simulink model "First_Model"  (R2021b)
settings: Solver=VariableStepDiscrete  StartTime=0.0  StopTime=200  MaxStep=inf  RelTol=1e-3
undefined symbols (not defined in the file): f, m, n
settings Model: Creator=david  LastModifiedBy=andry
settings SolverCC: AlgebraicLoopSolver=TrustRegion
settings DebuggingCC: SFMachineParentedDataDiag=warning

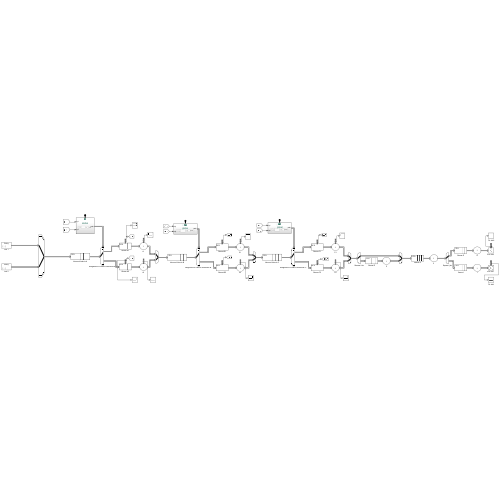
[thumbnail: Simulink's stored preview of the top-level diagram]
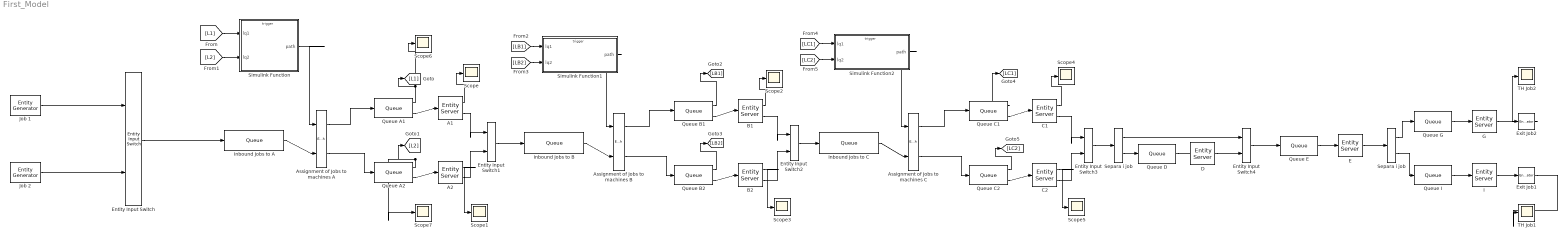
== system First_Model ==
  A1 : EntityServer  InputPortMessageModes=m  OutputPortMessageModes=n,m  Capacity=1  ServiceTimeValue=3  NumberEntitiesDeparted=on
      settings: OutputPortMap=o0,o9
  A2 : EntityServer  InputPortMessageModes=m  OutputPortMessageModes=n,m  Capacity=1  ServiceTimeValue=3  NumberEntitiesDeparted=on
      settings: OutputPortMap=o0,o9
  Assignment of Jobs to machines A : EntityOutputSwitch  InputPortMessageModes=m,m  OutputPortMessageModes=m,m  SwitchingCriterion=From control port  SwitchAttributeName=Attribute1
      settings: InputPortMap=u0,u1
  Assignment of Jobs to machines B : EntityOutputSwitch  InputPortMessageModes=m,m  OutputPortMessageModes=m,m  SwitchingCriterion=From control port  SwitchAttributeName=Attribute1
      settings: InputPortMap=u0,u1
  Assignment of Jobs to machines C : EntityOutputSwitch  InputPortMessageModes=m,m  OutputPortMessageModes=m,m  SwitchingCriterion=From control port  SwitchAttributeName=Attribute1
      settings: InputPortMap=u0,u1
  B1 : EntityServer  InputPortMessageModes=m  OutputPortMessageModes=n,m  Capacity=1  ServiceTimeValue=3  NumberEntitiesDeparted=on
      settings: OutputPortMap=o0,o9
  B2 : EntityServer  InputPortMessageModes=m  OutputPortMessageModes=n,m  Capacity=1  ServiceTimeValue=3  NumberEntitiesDeparted=on
      settings: OutputPortMap=o0,o9
  C1 : EntityServer  InputPortMessageModes=m  OutputPortMessageModes=n,m  Capacity=1  ServiceTimeValue=4  NumberEntitiesDeparted=on
      settings: OutputPortMap=o0,o9
  C2 : EntityServer  InputPortMessageModes=m  OutputPortMessageModes=n,m  Capacity=1  ServiceTimeValue=4  NumberEntitiesDeparted=on
      settings: OutputPortMap=o0,o9
  D : EntityServer  InputPortMessageModes=m  OutputPortMessageModes=m  Capacity=1  ServiceTimeValue=7
  E : EntityServer  InputPortMessageModes=m  OutputPortMessageModes=m  Capacity=1  ServiceTimeValue=4
  Entity Input Switch : EntityInputSwitch  InputPortMessageModes=m,m  OutputPortMessageModes=m  SwitchingCriterion=From control port
  Entity Input Switch{1..4} (4 alike) : EntityInputSwitch  InputPortMessageModes=m,m  OutputPortMessageModes=m
  Exit Job1 : EntityTerminator  InputPortMessageModes=m  NumberEntitiesArrived=on
      settings: OutputPortMap=o0
  Exit Job2 : EntityTerminator  InputPortMessageModes=m  NumberEntitiesArrived=on
      settings: OutputPortMap=o0
  G : EntityServer  InputPortMessageModes=m  OutputPortMessageModes=m  Capacity=1  ServiceTimeValue=8
  I : EntityServer  InputPortMessageModes=m  OutputPortMessageModes=m  Capacity=1  ServiceTimeValue=5
  Inbound Jobs to A : Queue  InputPortMessageModes=m  OutputPortMessageModes=m  Capacity=inf  PrioritySource=Attribute1
  Inbound Jobs to B : Queue  InputPortMessageModes=m  OutputPortMessageModes=m  Capacity=inf  PrioritySource=Attribute1
  Inbound Jobs to C : Queue  InputPortMessageModes=m  OutputPortMessageModes=m  Capacity=inf  PrioritySource=Attribute1
  Job 1 : EntityGenerator  OutputPortMessageModes=m  Period=50  GenerateAction=|  AttributeName=JobType  EntityType=Structured  EntityTypeName=Entity
      | f();
      | f1();
      | f2();
  Job 2 : EntityGenerator  OutputPortMessageModes=m  Period=50  GenerateAction=f();  AttributeName=JobType  AttributeInitialValue=2  EntityType=Structured  EntityTypeName=Entity
  Queue A1 : Queue  InputPortMessageModes=m  OutputPortMessageModes=n,m  AverageQueueLength=on
      settings: OutputPortMap=o3,o5
  Queue A2 : Queue  InputPortMessageModes=m  OutputPortMessageModes=n,m  AverageQueueLength=on
      settings: OutputPortMap=o3,o5
  Queue B1 : Queue  InputPortMessageModes=m  OutputPortMessageModes=n,m  NumberEntitiesDeparted=on
      settings: OutputPortMap=o0,o5
  Queue B2 : Queue  InputPortMessageModes=m  OutputPortMessageModes=n,m  NumberEntitiesDeparted=on
      settings: OutputPortMap=o0,o5
  Queue C1 : Queue  InputPortMessageModes=m  OutputPortMessageModes=n,m  AverageQueueLength=on
      settings: OutputPortMap=o3,o5
  Queue C2 : Queue  InputPortMessageModes=m  OutputPortMessageModes=n,m  AverageQueueLength=on
      settings: OutputPortMap=o3,o5
  Queue D : Queue  InputPortMessageModes=m  OutputPortMessageModes=m
  Queue E : Queue  InputPortMessageModes=m  OutputPortMessageModes=m
  Queue G : Queue  InputPortMessageModes=m  OutputPortMessageModes=m
  Queue I : Queue  InputPortMessageModes=m  OutputPortMessageModes=m
  Scope{,1..7} (8 alike) : Scope
  Separa i job : EntityOutputSwitch  InputPortMessageModes=m  OutputPortMessageModes=m,m  SwitchingCriterion=From attribute  SwitchAttributeName=JobType
  "Separa i job " : EntityOutputSwitch  InputPortMessageModes=m  OutputPortMessageModes=m,m  SwitchingCriterion=From attribute  SwitchAttributeName=JobType
  Simulink Function : Subsystem  TreatAsAtomicUnit=on
  Simulink Function1 : Subsystem  TreatAsAtomicUnit=on
  Simulink Function2 : Subsystem  TreatAsAtomicUnit=on
  TH Job1 : Scope
  TH Job2 : Scope
  wires:
  Job 2/1 -> Entity Input Switch/2
  Entity Input Switch/1 -> Inbound Jobs to A/1
  Queue A2/2 -> A2/1
  Queue A1/2 -> A1/1
  Entity Input Switch1/1 -> Inbound Jobs to B/1
  A1/2 -> Entity Input Switch1/1
  A2/2 -> Entity Input Switch1/2
  Inbound Jobs to B/1 -> Assignment of Jobs to machines B/2
  Queue B1/2 -> B1/1
  Queue B2/2 -> B2/1
  Assignment of Jobs to machines B/1 -> Queue B1/1
  Assignment of Jobs to machines B/2 -> Queue B2/1
  B1/2 -> Entity Input Switch2/1
  B2/2 -> Entity Input Switch2/2
  Inbound Jobs to C/1 -> Assignment of Jobs to machines C/2
  Assignment of Jobs to machines C/1 -> Queue C1/1
  Assignment of Jobs to machines C/2 -> Queue C2/1
  Queue C1/2 -> C1/1
  Queue C2/2 -> C2/1
  Entity Input Switch2/1 -> Inbound Jobs to C/1
  C1/2 -> Entity Input Switch3/1
  C2/2 -> Entity Input Switch3/2
  Entity Input Switch3/1 -> Separa i job/1
  Separa i job/2 -> Queue D/1
  Queue D/1 -> D/1
  Queue E/1 -> E/1
  Separa i job/1 -> Entity Input Switch4/1
  D/1 -> Entity Input Switch4/2
  Entity Input Switch4/1 -> Queue E/1
  E/1 -> "Separa i job "/1
  "Separa i job "/1 -> Queue G/1
  "Separa i job "/2 -> Queue I/1
  Queue G/1 -> G/1
  Queue I/1 -> I/1
  G/1 -> Exit Job2/1
  I/1 -> Exit Job1/1
  Exit Job1/1 -> TH Job1/1
  Exit Job2/1 -> TH Job2/1
  Inbound Jobs to A/1 -> Assignment of Jobs to machines A/2
  Assignment of Jobs to machines A/1 -> Queue A1/1
  Assignment of Jobs to machines A/2 -> Queue A2/1
  Queue A1/1 -> Scope6/1, [L1]
  Queue A2/1 -> Scope7/1, [L2]
  [L1] -> Simulink Function/1(lq1)
  [L2] -> Simulink Function/2(lq2)
  Simulink Function/1(path) -> Assignment of Jobs to machines A/1
  A1/1 -> Scope/1
  A2/1 -> Scope1/1
  Queue B1/1 -> [LB1]
  Queue B2/1 -> [LB2]
  Simulink Function1/1(path) -> Assignment of Jobs to machines B/1
  [LB1] -> Simulink Function1/1(lq1)
  [LB2] -> Simulink Function1/2(lq2)
  B1/1 -> Scope2/1
  B2/1 -> Scope3/1
  Queue C1/1 -> [LC1]
  Queue C2/1 -> [LC2]
  [LC1] -> Simulink Function2/1(lq1)
  [LC2] -> Simulink Function2/2(lq2)
  Simulink Function2/1(path) -> Assignment of Jobs to machines C/1
  C1/1 -> Scope4/1
  C2/1 -> Scope5/1
  Job 1/1 -> Entity Input Switch/1

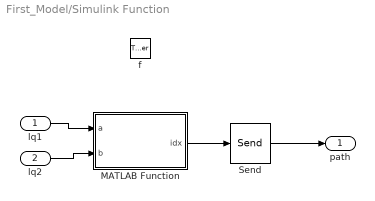
== system First_Model/Simulink Function ==
  lq1 : Inport
  lq2 : Inport  Port=2
  f : TriggerPort  TriggerType=function-call  IsSimulinkFunction=on  FunctionName=f  VariantControl=(inherit)
  MATLAB Function : MATLAB Function  TreatAsAtomicUnit=on
  Send : Send  OutputPortMessageModes=m
  path : Outport
  wires:
  lq1/1 -> MATLAB Function/1(a)
  lq2/1 -> MATLAB Function/2(b)
  MATLAB Function/1(idx) -> Send/1
  Send/1 -> path/1

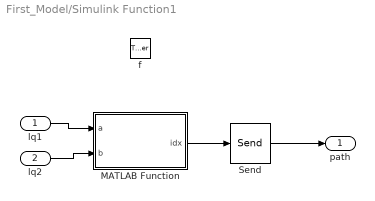
== system First_Model/Simulink Function1 ==
  lq1 : Inport
  lq2 : Inport  Port=2
  f : TriggerPort  TriggerType=function-call  IsSimulinkFunction=on  FunctionName=f1  VariantControl=(inherit)
  MATLAB Function : MATLAB Function  TreatAsAtomicUnit=on
  Send : Send  OutputPortMessageModes=m
  path : Outport
  wires:
  lq1/1 -> MATLAB Function/1(a)
  lq2/1 -> MATLAB Function/2(b)
  MATLAB Function/1(idx) -> Send/1
  Send/1 -> path/1

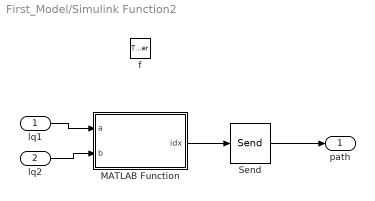
== system First_Model/Simulink Function2 ==
  lq1 : Inport
  lq2 : Inport  Port=2
  f : TriggerPort  TriggerType=function-call  IsSimulinkFunction=on  FunctionName=f2  VariantControl=(inherit)
  MATLAB Function : MATLAB Function  TreatAsAtomicUnit=on
  Send : Send  OutputPortMessageModes=m
  path : Outport
  wires:
  lq1/1 -> MATLAB Function/1(a)
  lq2/1 -> MATLAB Function/2(b)
  MATLAB Function/1(idx) -> Send/1
  Send/1 -> path/1

== matlab function First_Model/Simulink Function/MATLAB Function ==
  data: a input; idx output; b input

 function idx = fcn(a,b)
 
 [~, idx] = min([a,b]);

== matlab function First_Model/Simulink Function2/MATLAB Function ==
  data: a input; idx output; b input
function idx = fcn(a,b)

[~, idx] = min([a,b]);

== matlab function First_Model/Simulink Function1/MATLAB Function ==
  data: a input; idx output; b input
function idx = fcn(a,b)

[~, idx] = min([a,b]);
